simulink model "FourierTransform"  (R2018b)
settings: Solver=VariableStepAuto  StartTime=0.0  StopTime=10  RelTol=1e-3
libraries: powerlib x26, simulink x2, powerlib_meascontrol x2
settings Model: Creator=assia  LastModifiedBy=assia

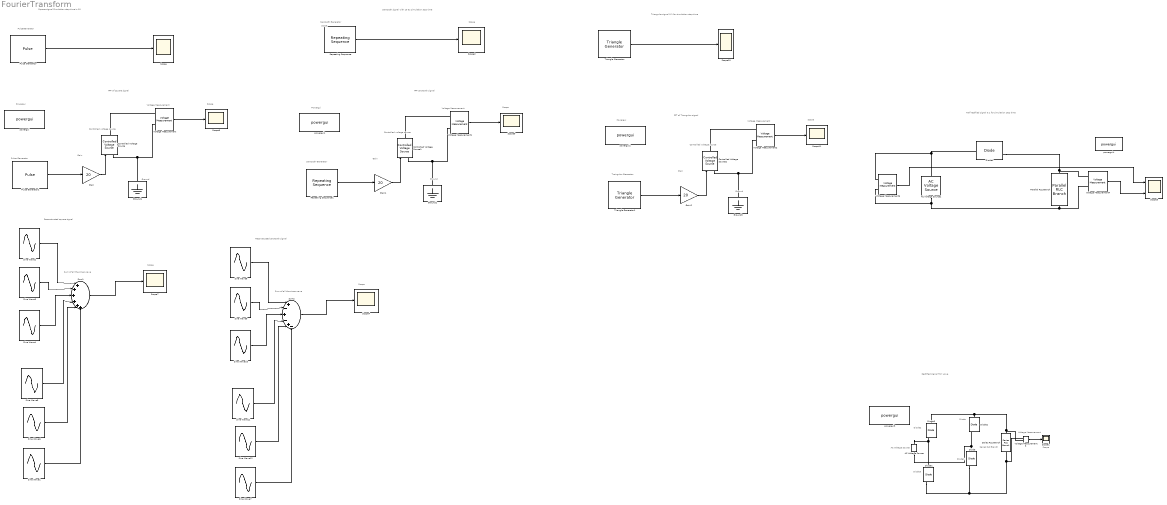
== system FourierTransform ==
  note: FFT of Triangular signal
  note: Triangular signal
      | 0.1 for simulation stop time
  note: FFT sawtooth signal
  note: Sawtooth signal
      | with 10 as simulation stop time
  note: FFT of square signal
  note: Reconstructed square signal
  note: Square signal
      | Simulation stop time is 10
  note: Scope
  note: Sawtooth Generator
  note: scope
  note: PulseGenerator
  note: Scope
  note: Voltage Measurement
  note: Pulse Generator
  note: Gain
  note: Powergui
  note: Ground
  note: Scope
  note: Sum of all the sines wave
  note: Controlled voltage source
  note: Controlled voltage source
  note: Sawtooth Generator
  note: Powergui
  note: Ground
  note: Gain
  note: Voltage Measurement
  note: Scope
  note: Controlled voltage source
  note: Gain
  note: Powergui
  note: Traingular Generator
  note: Scope
  note: Ground
  note: Voltage Measurement
  note: Half rectified signal
      | 0.1 for simulation stop time
  note: Diode2
  note: AC Voltage Source
  note: Series RLC Branch
  note: Diode
  note: Diode3
  note: Scope
  note: Voltage Measurement
  note: Rectified signal Full wave
  note: Diode1
  note: Scope
  note: Sum of all the sines wave
  note: Reconstructed sawtooth signal
  AC Voltage Source : powerlib/Electrical Sources/AC Voltage Source  Amplitude=10  Phase=0  Frequency=50  SampleTime=0  Measurements=None  BusType=swing  Pref=10e3  Qref=0  Qmin=-inf  Qmax=+inf
  AC Voltage Source1 : powerlib/Electrical Sources/AC Voltage Source  Amplitude=220  Phase=0  Frequency=50  SampleTime=0  Measurements=None  BusType=swing  Pref=10e3  Qref=0  Qmin=-inf  Qmax=+inf
  Controlled Voltage Source : powerlib/Electrical Sources/Controlled Voltage Source  Initialize=on  Source_Type=AC  Amplitude=0  Phase=0  Frequency=0  Measurements=None
  Controlled Voltage Source1 : powerlib/Electrical Sources/Controlled Voltage Source  Initialize=on  Source_Type=AC  Amplitude=0  Phase=0  Frequency=0  Measurements=None
  Controlled Voltage Source2 : powerlib/Electrical Sources/Controlled Voltage Source  Initialize=on  Source_Type=AC  Amplitude=0  Phase=0  Frequency=0  Measurements=None
  Diode{,1..3} (4 alike) : powerlib/Power Electronics/Diode  Ron=0.001  Lon=0  Vf=0.8  IC=0  UseSnubber=0  Rs=500  Cs=250e-9  Measurements=on
  Diode4 : powerlib/Power Electronics/Diode  Ron=0.001  Lon=0  Vf=0  IC=0  UseSnubber=0  Rs=inf  Cs=inf  Measurements=on
  Gain : Gain  Gain=20
  Gain1 : Gain  Gain=20
  Gain2 : Gain  Gain=20
  Ground1 : powerlib/Elements/Ground  LConnTagsString=a
  Ground2 : powerlib/Elements/Ground  LConnTagsString=a
  Ground3 : powerlib/Elements/Ground  LConnTagsString=a
  Parallel RLC Branch : powerlib/Elements/Parallel RLC Branch  LConnTagsString=a  RConnTagsString=__new0  BranchType=R  Resistance=1000  Inductance=1e-3  SetiL0=off  InitialCurrent=0  Capacitance=1e-6  Setx0=off  InitialVoltage=0  Measurements=None
  Pulse Generator : DiscretePulseGenerator  Period=10  SampleTime=5
  Pulse Generator1 : DiscretePulseGenerator  Period=5  SampleTime=5
  Repeating Sequence : simulink/Sources/Repeating Sequence  rep_seq_t=[0 2]  rep_seq_y=[0 2]
  Repeating Sequence1 : simulink/Sources/Repeating Sequence  rep_seq_t=[0 2]  rep_seq_y=[0 2]
  Scope{,1..2,4,7..11} (9 alike) : Scope
  Scope3 : Scope  NumInputPorts=2
  Series RLC Branch : powerlib/Elements/Series RLC Branch  LConnTagsString=__new0  RConnTagsString=__new0  BranchType=R  Resistance=100  Inductance=1e-3  SetiL0=off  InitialCurrent=0  Capacitance=1e-6  Setx0=off  InitialVoltage=0  Measurements=None
  Sine Wave1 : Sin  Amplitude=1/11  Frequency=11*2*pi  SampleTime=0
  Sine Wave10 : Sin  Amplitude=1/4  Frequency=3  SampleTime=0
  Sine Wave11 : Sin  Amplitude=1/5  Frequency=4  SampleTime=0
  Sine Wave12 : Sin  Amplitude=1/6  Frequency=5  SampleTime=0
  Sine Wave2 : Sin  Frequency=1*2*pi  SampleTime=0
  Sine Wave3 : Sin  Amplitude=1/3  Frequency=3*2*pi  SampleTime=0
  Sine Wave4 : Sin  Amplitude=1/5  Frequency=5*2*pi  SampleTime=0
  Sine Wave5 : Sin  Amplitude=1/7  Frequency=7*2*pi  SampleTime=0
  Sine Wave6 : Sin  Amplitude=1/9  Frequency=9*2*pi  SampleTime=0
  Sine Wave7 : Sin  Amplitude=1/7  Frequency=6  SampleTime=0
  Sine Wave8 : Sin  Amplitude=1/2  SampleTime=0
  Sine Wave9 : Sin  Amplitude=1/3  Frequency=2  SampleTime=0
  Sum1 : Sum  Inputs=|++++++
  Sum2 : Sum  Inputs=|+-+-+-
  Triangle Generator : powerlib_meascontrol/Pulse & Signal Generators/Triangle Generator  Freq=1e3  Phase=90  Ts=0
  Triangle Generator1 : powerlib_meascontrol/Pulse & Signal Generators/Triangle Generator  Freq=1e3  Phase=90  Ts=0
  Voltage Measurement{,1..4,6} (6 alike) : powerlib/Measurements/Voltage Measurement  PhasorSimulation=off  OutputType=Complex  PSBequivalent=0
  powergui : powerlib/powergui  Priority=1  SimulationMode=Continuous  SampleTime=50e-6  frequency=60  Iterations=50  frequencyindice=50  Pbase=100e6  ErrMax=1e-4  UnitsV=kV  UnitsW=MW  buscounter=0  FunctionMessages=off  echomessages=off  EnableUseOfTLC=off  CurrentSourceSwitches=off  DisableSnubberDevices=off  DisableRonSwitches=off  DisableVfSwitches=off  DisplayEquations=off  SolverType=Tustin/Backward Euler (TBE)  Interpol=off  ExternalGateDelay=off  methode=off  Ts=100  x0status=blocks  SPID=on  SwTol=0  HookPort=off  RestoreLinks=warning  ResistiveCurrentMeasurement=off  Frange=[0:2:500]  Ylog=off  Xlog=on  ShowGrid=off  save=off  variable=ZData  structure=Square  ZoomFFT=off  StartTime=0  cycles=400  DisplayStyle=1  fundamental=50  FreqAxis=off  MaxFrequency=1000  frequencyindicesteady=1  RmsSteady=1  display=off
  powergui1 : powerlib/powergui  Priority=1  SimulationMode=Continuous  SampleTime=50e-6  frequency=60  Iterations=50  frequencyindice=0  Pbase=100e6  ErrMax=1e-4  UnitsV=kV  UnitsW=MW  buscounter=0  FunctionMessages=off  echomessages=off  EnableUseOfTLC=off  CurrentSourceSwitches=off  DisableSnubberDevices=off  DisableRonSwitches=off  DisableVfSwitches=off  DisplayEquations=off  SolverType=Tustin/Backward Euler (TBE)  Interpol=off  ExternalGateDelay=off  methode=off  Ts=100  x0status=blocks  SPID=on  SwTol=0  HookPort=off  RestoreLinks=warning  ResistiveCurrentMeasurement=off  Frange=[0:2:500]  Ylog=off  Xlog=on  ShowGrid=off  save=off  variable=ZData  structure=Saw  ZoomFFT=on  StartTime=0  cycles=400  DisplayStyle=1  fundamental=50  FreqAxis=off  MaxFrequency=1000  frequencyindicesteady=1  RmsSteady=1  display=off
  powergui2 : powerlib/powergui  Priority=1  SimulationMode=Continuous  SampleTime=50e-6  frequency=60  Iterations=50  frequencyindice=0  Pbase=100e6  ErrMax=1e-4  UnitsV=kV  UnitsW=MW  buscounter=0  FunctionMessages=off  echomessages=off  EnableUseOfTLC=off  CurrentSourceSwitches=off  DisableSnubberDevices=off  DisableRonSwitches=off  DisableVfSwitches=off  DisplayEquations=off  SolverType=Tustin/Backward Euler (TBE)  Interpol=off  ExternalGateDelay=off  methode=off  Ts=100  x0status=blocks  SPID=on  SwTol=0  HookPort=off  RestoreLinks=warning  ResistiveCurrentMeasurement=off  Frange=[0:2:500]  Ylog=off  Xlog=on  ShowGrid=off  save=off  variable=ZData  structure=triangul  ZoomFFT=on  StartTime=0  cycles=1  DisplayStyle=1  fundamental=50  FreqAxis=off  MaxFrequency=1000  frequencyindicesteady=1  RmsSteady=1  display=off
  powergui3 : powerlib/powergui  Priority=1  SimulationMode=Continuous  SampleTime=50e-6  frequency=60  Iterations=50  frequencyindice=0  Pbase=100e6  ErrMax=1e-4  UnitsV=kV  UnitsW=MW  buscounter=0  FunctionMessages=off  echomessages=off  EnableUseOfTLC=off  CurrentSourceSwitches=off  DisableSnubberDevices=off  DisableRonSwitches=off  DisableVfSwitches=off  DisplayEquations=off  SolverType=Tustin/Backward Euler (TBE)  Interpol=off  ExternalGateDelay=off  methode=off  Ts=100  x0status=blocks  SPID=on  SwTol=0  HookPort=off  RestoreLinks=warning  ResistiveCurrentMeasurement=off  Frange=[0:2:500]  Ylog=off  Xlog=on  ShowGrid=off  save=off  variable=ZData  structure=rectified  ZoomFFT=on  StartTime=0  cycles=1  DisplayStyle=1  fundamental=50  FreqAxis=off  MaxFrequency=1000  frequencyindicesteady=1  RmsSteady=1  display=off
  powergui4 : powerlib/powergui  Priority=1  SimulationMode=Continuous  SampleTime=50e-6  frequency=60  Iterations=50  frequencyindice=60  Pbase=100e6  ErrMax=1e-4  UnitsV=kV  UnitsW=MW  buscounter=0  FunctionMessages=off  echomessages=off  EnableUseOfTLC=off  CurrentSourceSwitches=off  DisableSnubberDevices=off  DisableRonSwitches=off  DisableVfSwitches=off  DisplayEquations=off  SolverType=Tustin/Backward Euler (TBE)  Interpol=off  ExternalGateDelay=off  methode=off  Ts=100  x0status=blocks  SPID=on  SwTol=0  HookPort=off  RestoreLinks=warning  ResistiveCurrentMeasurement=off  Frange=[0:2:500]  Ylog=off  Xlog=on  ShowGrid=off  save=off  variable=ZData  structure=halfR  ZoomFFT=on  StartTime=0.0  cycles=1  DisplayStyle=1  fundamental=60  FreqAxis=off  MaxFrequency=1000  frequencyindicesteady=1  RmsSteady=1  display=off
  wires:
  Repeating Sequence/1 -> Scope2/1
  Pulse Generator/1 -> Scope/1
  Voltage Measurement/1 -> Scope8/1
  Sine Wave4/1 -> Sum1/3
  Sine Wave1/1 -> Sum1/6
  Sine Wave6/1 -> Sum1/5
  Sine Wave2/1 -> Sum1/1
  Gain/1 -> Controlled Voltage Source/1
  Sum1/1 -> Scope7/1
  Sine Wave3/1 -> Sum1/2
  Sine Wave5/1 -> Sum1/4
  Pulse Generator1/1 -> Gain/1
  Gain1/1 -> Controlled Voltage Source1/1
  Voltage Measurement1/1 -> Scope9/1
  Repeating Sequence1/1 -> Gain1/1
  Triangle Generator/1 -> Scope10/1
  Triangle Generator1/1 -> Gain2/1
  Gain2/1 -> Controlled Voltage Source2/1
  Voltage Measurement2/1 -> Scope11/1
  Voltage Measurement6/1 -> Scope3/1
  Voltage Measurement4/1 -> Scope3/2
  Voltage Measurement3/1 -> Scope1/1
  Sine Wave12/1 -> Sum2/5
  Sine Wave7/1 -> Sum2/6
  Sine Wave9/1 -> Sum2/2
  Sine Wave8/1 -> Sum2/1
  Sum2/1 -> Scope4/1
  Sine Wave10/1 -> Sum2/3
  Sine Wave11/1 -> Sum2/4
  connections:
  Voltage Measurement/LConn2 -- Controlled Voltage Source/LConn1 -- Ground1/LConn1
  Controlled Voltage Source/RConn1 -- Voltage Measurement/LConn1
  Voltage Measurement1/LConn2 -- Controlled Voltage Source1/LConn1 -- Ground2/LConn1
  Controlled Voltage Source1/RConn1 -- Voltage Measurement1/LConn1
  Voltage Measurement2/LConn2 -- Controlled Voltage Source2/LConn1 -- Ground3/LConn1
  Controlled Voltage Source2/RConn1 -- Voltage Measurement2/LConn1
  AC Voltage Source1/RConn1 -- Voltage Measurement6/LConn1 -- Diode4/LConn1
  Parallel RLC Branch/LConn1 -- Diode4/RConn1 -- Voltage Measurement4/LConn1
  Parallel RLC Branch/RConn1 -- Voltage Measurement6/LConn2 -- AC Voltage Source1/LConn1 -- Voltage Measurement4/LConn2
  Diode3/RConn1 -- Diode1/LConn1 -- AC Voltage Source/RConn1
  Series RLC Branch/LConn1 -- Voltage Measurement3/LConn2 -- Diode2/LConn1 -- Diode3/LConn1
  Series RLC Branch/RConn1 -- Voltage Measurement3/LConn1 -- Diode/RConn1 -- Diode1/RConn1
  Diode/LConn1 -- AC Voltage Source/LConn1 -- Diode2/RConn1
